simulink library "rtc"  (R2015a)
settings: Solver=ode45  SolverMode=SingleTasking  StartTime=0.0  StopTime=10.0  RelTol=1e-3
settings Model: Creator=uvs  LastModifiedBy=uvs
settings DataIOCC: SignalLoggingSaveFormat=ModelDataLogs
settings OptimizationCC: BlockReduction=off  BooleanDataType=off
settings DebuggingCC: SaveWithParameterizedLinksMsg=none  UnderspecifiedInitializationDetection=Classic  MergeDetectMultiDrivingBlocksExec=none  SignalResolutionControl=TryResolveAllWithWarning  MultiTaskCondExecSysMsg=none  StrictBusMsg=None
settings HardwareCC: TargetUnknown=on

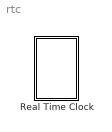
== system rtc ==
  Real Time Clock : Subsystem

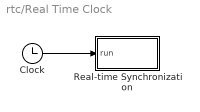
== system rtc/Real Time Clock ==
  Clock : Clock
  Real-time Synchronization : Subsystem
  wires:
  Clock/1 -> Real-time Synchronization/1(run)

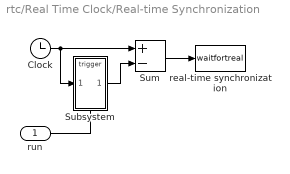
== system rtc/Real Time Clock/Real-time Synchronization ==
  run : Inport
  Clock : Clock
  Subsystem : Subsystem  TreatAsAtomicUnit=on
  Sum : Sum  Inputs=+-  SaturateOnIntegerOverflow=on  InputSameDT=on  OutDataTypeStr=Inherit: Same as first input
  real-time synchronization : MATLABFcn  MATLABFcn=waitfortreal  OutputDimensions=0
  wires:
  run/1 -> Subsystem/Trigger
  Sum/1 -> real-time synchronization/1
  Subsystem/1(Out) -> Sum/2
  Clock/1 -> Sum/1, Subsystem/1(In)

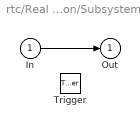
== system rtc/Real Time Clock/Real-time Synchronization/Subsystem ==
  In : Inport
  Trigger : TriggerPort
  Out : Outport  InitialOutput=0
  wires:
  In/1 -> Out/1
